simulink model "FeedforwardFeedbackControl"  (R2024b)
settings: Solver=VariableStepAuto  StartTime=0.0  StopTime=10.0  RelTol=1e-3
undefined symbols (not defined in the file): Kc, Kp
settings Model: Creator=emersonhall  LastModifiedBy=emersonhall

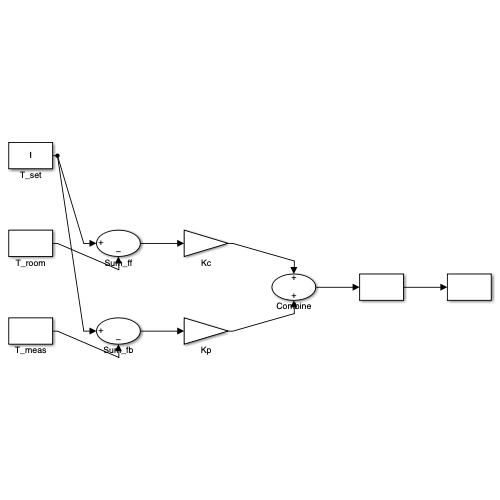
[thumbnail: Simulink's stored preview of the top-level diagram]
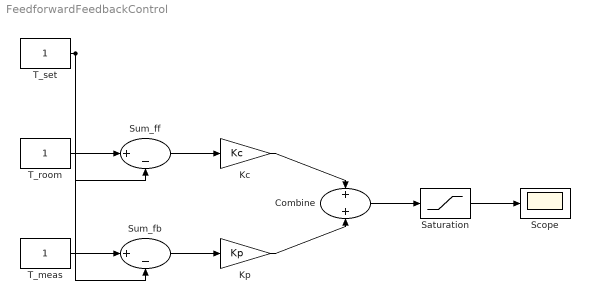
== system FeedforwardFeedbackControl ==
  Combine : Sum
  Kc : Gain  Gain=Kc
  Kp : Gain  Gain=Kp
  Saturation : Saturate
  Scope : Scope
  Sum_fb : Sum  Inputs=|+-
  Sum_ff : Sum  Inputs=|+-
  T_meas : Constant
  T_room : Constant
  T_set : Constant
  wires:
  T_set/1 -> Sum_ff/1, Sum_fb/1
  T_room/1 -> Sum_ff/2
  T_meas/1 -> Sum_fb/2
  Sum_ff/1 -> Kc/1
  Sum_fb/1 -> Kp/1
  Kc/1 -> Combine/1
  Kp/1 -> Combine/2
  Combine/1 -> Saturation/1
  Saturation/1 -> Scope/1
